simulink model "st400w_ce"  (R2016b)
settings: Solver=ode15s  StartTime=0.0  StopTime=20000  MaxStep=Ts*5  RelTol=1e-2  EnableMultiTasking=on
StopFcn:
  | %qpOASES_sequence('c');
values from neighbouring files (symbols this model uses):
  Ao = Ad    [cold_end_script.m]    (also in observateur.m = [A Bunc; zeros(size(Bunc,2),size(A,1)), eye(size(Bunc,2))])
  Aoe = Ao-L*Co    [cold_end_script.m]    (also in observateur.m)
  Boe = [Bo-L*Do Fo-L*Go L]    [cold_end_script.m]    (also in observateur.m = [Bo-L*Do L])
  Co = Cd    [cold_end_script.m]    (also in observateur.m = [C Dunc])
  Coe = eye(length(Ao))    [cold_end_script.m]    (also in observateur.m)
  Do = Dd    [cold_end_script.m]    (also in observateur.m = D)
  Doe = zeros(size(Coe*Boe))    [cold_end_script.m]    (also in observateur.m)
  Go = Gd    [cold_end_script.m]
  ini = 0    [cold_end_script.m]
  mpc = cstr_func(mpc)    [cold_end_script.m]    (also in mpc_control.m = def_pb_mpc(u_t,w_t,x_t,y_ref_t,u_ref_t,mpc))
  Tp = 5    [cold_end_script.m]
undefined symbols (not defined in the file or in its folder): mpc_control
libraries: simCryogenics_lib x36, nesl_utility x24
settings Model: Creator=FB229602  LastModifiedBy=trinhvv-admin
settings SolverCC: InitialStep=2.5
settings DataIOCC: LimitDataPoints=on  SaveFormat=Array
settings OptimizationCC: LifeSpan=inf
settings DebuggingCC: SFUnexpectedBacktrackingDiag=warning  SFNoUnconditionalDefaultTransitionDiag=warning  SFExecutionAtInitializationDiag=none
settings HardwareCC: ProdBitPerPointer=32  ProdBitPerSizeT=32  ProdBitPerPtrDiffT=32  ProdLargestAtomicFloat=None  ProdIntDivRoundTo=Undefined  ProdEndianess=Unspecified  ProdWordSize=32  ProdHWDeviceType=32-bit Generic
settings ModelReferenceCC: PropagateSignalLabelsOutOfModel=off
settings GRTTargetCC: TargetLangStandard=C89/C90 (ANSI)  GeneratePreprocessorConditionals=Disable all
settings ConfigComp: CovMetricSettings=dw  CovHtmlReporting=on  CovSaveCumulativeToWorkspaceVar=on  CovSaveSingleToWorkspaceVar=on  CovExternalEMLEnable=off
settings SimscapeCC: SimscapeLogType=all  SimscapeLogLimitData=off

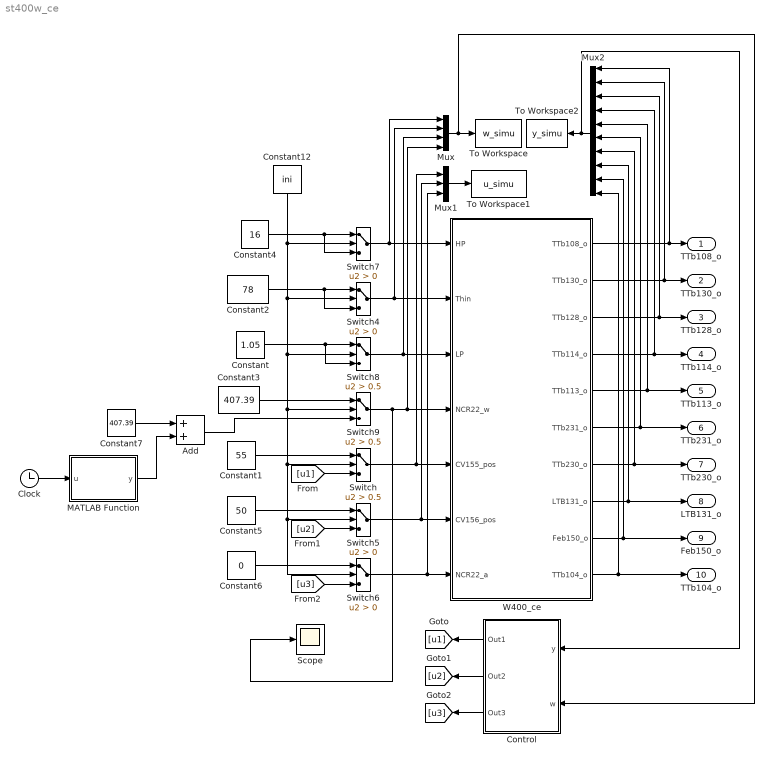
== system st400w_ce ==
  Add : Sum
  Clock : Clock
  Constant : Constant  Value=1.05
  Constant1 : Constant  Value=55
  Constant12 : Constant  Value=ini
  Constant2 : Constant  Value=78
  Constant3 : Constant  Value=407.39
  Constant4 : Constant  Value=16
  Constant5 : Constant  Value=50
  Constant6 : Constant  Value=0
  Constant7 : Constant  Value=407.39
  Control : Subsystem
  MATLAB Function : MATLAB Function  TreatAsAtomicUnit=on
  Mux : Mux
  Mux1 : Mux  Inputs=3
  Mux2 : Mux  Inputs=10
  Scope : Scope
  Switch : Switch  Criteria=u2 > Threshold  Threshold=0.5
  Switch{4..7} (4 alike) : Switch  Criteria=u2 > Threshold
  Switch8 : Switch  Criteria=u2 > Threshold  Threshold=0.5
  Switch9 : Switch  Criteria=u2 > Threshold  Threshold=0.5
  To Workspace : ToWorkspace  VariableName=w_simu  SampleTime=-1
      settings: Save2DSignal=2-D array (concatenate along first dimension)
  To Workspace1 : ToWorkspace  VariableName=u_simu  SampleTime=-1
      settings: Save2DSignal=2-D array (concatenate along first dimension)
  To Workspace2 : ToWorkspace  VariableName=y_simu  SampleTime=-1
      settings: Save2DSignal=2-D array (concatenate along first dimension)
  W400_ce : Subsystem
  TTb108_o : Outport
  TTb130_o : Outport  Port=2
  TTb128_o : Outport  Port=3
  TTb114_o : Outport  Port=4
  TTb113_o : Outport  Port=5
  TTb231_o : Outport  Port=6
  TTb230_o : Outport  Port=7
  LTB131_o : Outport  Port=8
  Feb150_o : Outport  Port=9
  TTb104_o : Outport  Port=10
  wires:
  Switch8/1 -> Mux/3, W400_ce/3(LP)
  Switch7/1 -> Mux/1, W400_ce/1(HP)
  Switch5/1 -> Mux1/2, W400_ce/6(CV156_pos)
  Switch/1 -> Mux1/1, W400_ce/5(CV155_pos)
  Switch6/1 -> Mux1/3, W400_ce/7(NCR22_a)
  W400_ce/1(TTb108_o) -> Mux2/1, TTb108_o/1
  W400_ce/2(TTb130_o) -> Mux2/2, TTb130_o/1
  W400_ce/3(TTb128_o) -> Mux2/3, TTb128_o/1
  W400_ce/4(TTb114_o) -> Mux2/4, TTb114_o/1
  W400_ce/5(TTb113_o) -> Mux2/5, TTb113_o/1
  W400_ce/6(TTb231_o) -> Mux2/6, TTb231_o/1
  W400_ce/7(TTb230_o) -> Mux2/7, TTb230_o/1
  W400_ce/8(LTB131_o) -> Mux2/8, LTB131_o/1
  W400_ce/9(Feb150_o) -> Mux2/9, Feb150_o/1
  Switch9/1 -> Scope/1, W400_ce/4(NCR22_w), Mux/4
  W400_ce/10(TTb104_o) -> TTb104_o/1, Mux2/10
  Switch4/1 -> Mux/2, W400_ce/2(Thin)
  Constant6/1 -> Switch6/1
  Constant1/1 -> Switch/1
  Constant5/1 -> Switch5/1
  Constant12/1 -> Switch6/2, Switch5/2, Switch/2, Switch9/2, Switch8/2, Switch4/2, Switch7/2
  Constant2/1 -> Switch4/3, Switch4/1
  Constant4/1 -> Switch7/3, Switch7/1
  Control/1(Out1) -> [u1]
  Control/2(Out2) -> [u2]
  Control/3(Out3) -> [u3]
  Constant/1 -> Switch8/3, Switch8/1
  Add/1 -> Switch9/3
  Mux1/1 -> To Workspace1/1
  Mux/1 -> Control/2(w), To Workspace/1
  Mux2/1 -> Control/1(y), To Workspace2/1
  [u1] -> Switch/3
  [u2] -> Switch5/3
  [u3] -> Switch6/3
  Constant3/1 -> Switch9/1
  Constant7/1 -> Add/1
  MATLAB Function/1(y) -> Add/2
  Clock/1 -> MATLAB Function/1(u)

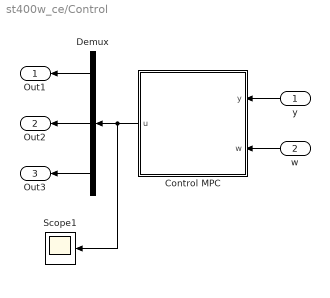
== system st400w_ce/Control ==
  y : Inport
  w : Inport  Port=2
  Control MPC : Subsystem
  Demux : Demux  Outputs=3
  Scope1 : Scope
  Out1 : Outport
  Out2 : Outport  Port=2
  Out3 : Outport  Port=3
  wires:
  Demux/1 -> Out1/1
  Demux/2 -> Out2/1
  Demux/3 -> Out3/1
  Control MPC/1(u) -> Scope1/1, Demux/1
  y/1 -> Control MPC/1(y)
  w/1 -> Control MPC/2(w)

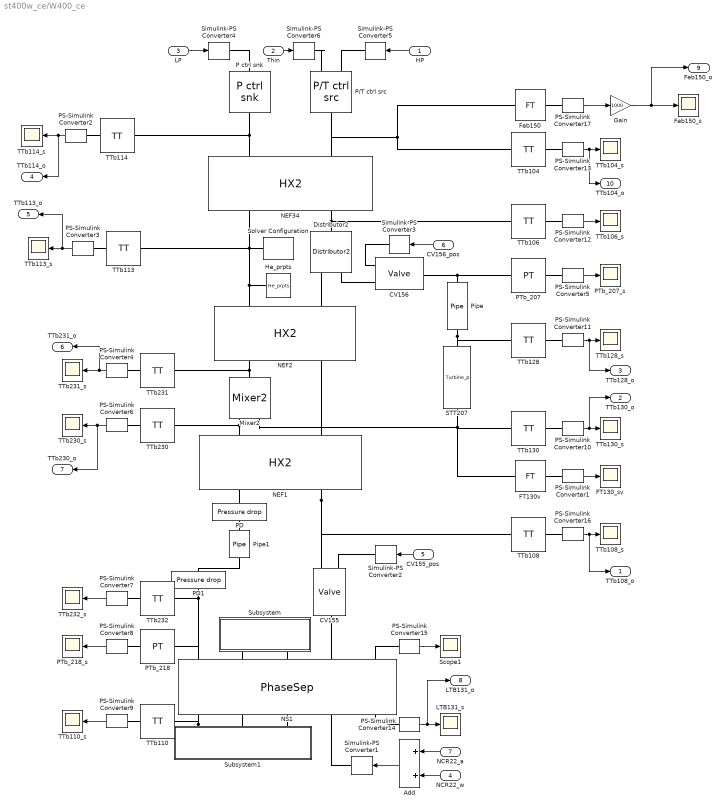
== system st400w_ce/W400_ce ==
  HP : Inport
  Thin : Inport  Port=2
  LP : Inport  Port=3
  NCR22_w : Inport  Port=4
  CV155_pos : Inport  Port=5
  CV156_pos : Inport  Port=6
  NCR22_a : Inport  Port=7
  Add : Sum
  CV155 : simCryogenics_lib/Elements/Valve  CVmax=0.55  ControlInputMin=0  ControlInputMax=100  Xt=0.86  Rv=10  lin_v=0  lim_v=0  K=2.4e-5 m^1.50000*kg^0.50000/s/bar^0.50000  Cmd_specify=off  Cmd_priority=High  Cmd=0  gamma_specify=off  gamma_priority=High  gamma=0  rho_specify=off  rho_priority=High  rho=0 kg/m^3  Xc_specify=off  Xc_priority=High  Xc=0  X_specify=off  X_priority=High  X=0  Y_specify=off  Y_priority=High  Y=0  CV_specify=off  CV_priority=High  CV=0
  CV156 : simCryogenics_lib/Elements/Valve  CVmax=Cv  ControlInputMin=0  ControlInputMax=100  Xt=0.86  Rv=Rv  lin_v=0  lim_v=0  K=2.4e-5 m^1.50000*kg^0.50000/s/bar^0.50000  Cmd_specify=off  Cmd_priority=High  Cmd=0  gamma_specify=off  gamma_priority=High  gamma=0  rho_specify=off  rho_priority=High  rho=0 kg/m^3  Xc_specify=off  Xc_priority=High  Xc=0  X_specify=off  X_priority=High  X=0  Y_specify=off  Y_priority=High  Y=0  CV_specify=off  CV_priority=High  CV=0
  Distributor2 : simCryogenics_lib/Elements/Distributor2
  FT130_sv : Scope
  FT130v : simCryogenics_lib/Sensors/FT
  Feb150 : simCryogenics_lib/Sensors/FT
  Feb150_s : Scope
  Gain : Gain  Gain=1000
  He_prpts : simCryogenics_lib/Utilities/He_prpts  P_min=0.25 bar  P_max=18 bar  T_min=2 K  T_max=80 K  N=100  Mol=4.0026 * 10 ^ (- 3) kg/mol
  LTB131_s : Scope
  Mixer2 : simCryogenics_lib/Elements/Mixer2
  NEF1 : simCryogenics_lib/Elements/HX2  N=3  Vh=2.3e-3 m^3  Vc=2.3e-3 m^3  M=13 kg  Kh=0.6 s*bar/kg  Kc=0.35 s*bar/kg  h=H1 J/s/K  Th0=10 K  Ph0=16 bar  Mh0=0.037 kg/s  Tc0=4.5 K  Pc0=1.1 bar  Mc0=0.037 kg/s
  NEF2 : simCryogenics_lib/Elements/HX2  N=3  Vh=0.02 m^3  Vc=0.03 m^3  M=100 kg  Kh=0.6 s*bar/kg  Kc=0.35 s*bar/kg  h=H2 J/s/K  Th0=20 K  Ph0=16 bar  Mh0=0.037 kg/s  Tc0=10 K  Pc0=1.1 bar  Mc0=0.037 kg/s
  NEF34 : simCryogenics_lib/Elements/HX2  N=3  Vh=0.1 m^3  Vc=0.3 m^3  M=400 kg  Kh=0.6 s*bar/kg  Kc=0.35 s*bar/kg  h=H3 J/s/K  Th0=80 K  Ph0=16 bar  Mh0=0.037 kg/s  Tc0=20 K  Pc0=1.1 bar  Mc0=0.037 kg/s
  NS1 : simCryogenics_lib/Elements/PhaseSep  Ideal1=1  DeltaT1=0.05 K  N1=10  h1=400 W/K  Ideal2=1  DeltaT2=0.05 K  N2=10  h2=400 W/K  hmax=0.8 m  S=0.1662 m^2  P0=1.2 bar  h0=62  T0=4.5 K
  P ctrl snk : simCryogenics_lib/Sources_Sinks/P ctrl snk
  P/T ctrl src : simCryogenics_lib/Sources_Sinks/P//T ctrl src
  PD : simCryogenics_lib/Utilities/Pressure drop  K=0.01/0.03 s*bar/kg
  PD1 : simCryogenics_lib/Utilities/Pressure drop  K=0.0001/0.03 s*bar/kg
  PS-Simulink Converter{1..17} (17 alike) : nesl_utility/PS-Simulink Converter  PhysicalDomain=network_engine_domain  SubClassName=ps_output  LeftPortType=input  RightPortType=output  PseudoPeriodic=off  Frequencies=[]  Unit=1  AffineConversion=off
  PTb_207 : simCryogenics_lib/Sensors/PT
  PTb_207_s : Scope
  PTb_218 : simCryogenics_lib/Sensors/PT
  PTb_218_s : Scope
  Pipe : simCryogenics_lib/Elements/Pipe  Vol=0.05 m^3  Ideal=0  P0=14 bar  T0=22 K
  Pipe1 : simCryogenics_lib/Elements/Pipe  Vol=0.162*0.3 m^3  Ideal=0  P0=1.2 bar  T0=4.5 K
  STT207 : simCryogenics_lib/Elements/Turbine_p  A=5.4278e-06 m^2  D=0.022 m  Mass=0.02 kg  cst_eff=1  eta0=0.75  Tin0=20 K  Pin0=16 bar  Pout0=1.2 bar  N0=2500 1/s  Q0=0 W  v0=0  I=0 kg*m^2  gamma_specify=off  gamma_priority=High  gamma=0  C_specify=off  C_priority=High  C=0  Z_specify=off  Z_priority=High  Z=0  Cp_specify=off  Cp_priority=High  Cp=0 kJ/kg/K  Sin_specify=off  Sin_priority=High  Sin=0 kJ/kg  T_specify=off  T_priority=High  T=0 K  HoutIs_specify=off  HoutIs_priority=High  HoutIs=0 kJ/kg  u1_specify=off  u1_priority=High  u1=0 m/s  c1_specify=off  c1_priority=High  c1=0 m/s  v_specify=off  v_priority=High  v=0  eta_specify=off  eta_priority=High  eta=0  eta_var_specify=off  eta_var_priority=High  eta_var=0  N_specify=off  N_priority=High  N=0 rad/s  Q_specify=off  Q_priority=High  Q=0 W
  Scope1 : Scope
  Simulink-PS Converter{1,3..5} (4 alike) : nesl_utility/Simulink-PS Converter  PhysicalDomain=network_engine_domain  SubClassName=ps_input  LeftPortType=input  RightPortType=output  PseudoPeriodic=off  Frequencies=[]  NoiseDistribution=none  NoiseParameters=[]  Unit=1  AffineConversion=off  InputFiltering=off  SimscapeFilterOrder=1  InputFilterTimeConstant=1  UdotUserProvided=1
  Simulink-PS Converter2 : nesl_utility/Simulink-PS Converter  PhysicalDomain=network_engine_domain  SubClassName=ps_input  LeftPortType=input  RightPortType=output  PseudoPeriodic=off  Frequencies=[]  NoiseDistribution=none  NoiseParameters=[]  Unit=1  AffineConversion=off  InputFiltering=off  SimscapeFilterOrder=1  InputFilterTimeConstant=0.001  UdotUserProvided=1
  Simulink-PS Converter6 : nesl_utility/Simulink-PS Converter  PhysicalDomain=network_engine_domain  SubClassName=ps_input  LeftPortType=input  RightPortType=output  PseudoPeriodic=off  Frequencies=[]  NoiseDistribution=none  NoiseParameters=[]  Unit=1  AffineConversion=off  InputFiltering=off  SimscapeFilterOrder=1  InputFilterTimeConstant=0.001  UdotUserProvided=1
  Solver Configuration : nesl_utility/Solver Configuration  PhysicalDomain=network_engine_domain  SubClassName=solver  LeftPortType=input  RightPortType=generic  Accelerate=off  Tones=[]  Harmonics=[]  SimulateNoise=off  Profile=off  UseLocalSampling=off  EnableSwitchedLinearOptims=on  FrequencyDomain=off  UseCCode=off  RelTol=0.001  AbsTol=1e-06  MinStep=1e-09  ToWorkspace=off  RevertToSquareIcSolve=off  NumHomotopyIterations=100  PhasorMode=off  PhasorModeNumHarmonics=1  OverrideAbsTol=off  DoDC=off  ResidualTolerance=1e-09  UseLocalSolver=off  LocalSolverChoice=NE_BACKWARD_EULER_ADVANCER  LocalSolverSampleTime=5  DoFixedCost=off  MaxNonlinIter=3  MaxModeIter=2  LinearAlgebra=Sparse  DelaysMemoryBudget=1024  AutomaticFiltering=on  FilteringTimeConstant=0.001
  Subsystem : Subsystem
  Subsystem1 : Subsystem
  TTb{104,106,108,110,113..114,128,130,230..232} (11 alike) : simCryogenics_lib/Sensors/TT
  TTb104_s : Scope
  TTb106_s : Scope
  TTb108_s : Scope
  TTb110_s : Scope
  TTb113_s : Scope
  TTb114_s : Scope
  TTb128_s : Scope
  TTb130_s : Scope
  TTb230_s : Scope
  TTb231_s : Scope
  TTb232_s : Scope
  TTb108_o : Outport
  TTb130_o : Outport  Port=2
  TTb128_o : Outport  Port=3
  TTb114_o : Outport  Port=4
  TTb113_o : Outport  Port=5
  TTb231_o : Outport  Port=6
  TTb230_o : Outport  Port=7
  LTB131_o : Outport  Port=8
  Feb150_o : Outport  Port=9
  TTb104_o : Outport  Port=10
  wires:
  Gain/1 -> Feb150_o/1, Feb150_s/1
  CV155_pos/1 -> Simulink-PS Converter2/1
  HP/1 -> Simulink-PS Converter5/1
  Thin/1 -> Simulink-PS Converter6/1
  LP/1 -> Simulink-PS Converter4/1
  NCR22_w/1 -> Add/2
  NCR22_a/1 -> Add/1
  PS-Simulink Converter17/1 -> Gain/1
  PS-Simulink Converter16/1 -> TTb108_o/1, TTb108_s/1
  PS-Simulink Converter1/1 -> FT130_sv/1
  CV156_pos/1 -> Simulink-PS Converter3/1
  PS-Simulink Converter5/1 -> PTb_207_s/1
  PS-Simulink Converter12/1 -> TTb106_s/1
  PS-Simulink Converter11/1 -> TTb128_o/1, TTb128_s/1
  PS-Simulink Converter10/1 -> TTb130_o/1, TTb130_s/1
  PS-Simulink Converter9/1 -> TTb110_s/1
  PS-Simulink Converter8/1 -> PTb_218_s/1
  PS-Simulink Converter7/1 -> TTb232_s/1
  PS-Simulink Converter6/1 -> TTb230_o/1, TTb230_s/1
  PS-Simulink Converter4/1 -> TTb231_o/1, TTb231_s/1
  PS-Simulink Converter3/1 -> TTb113_o/1, TTb113_s/1
  PS-Simulink Converter2/1 -> TTb114_s/1, TTb114_o/1
  PS-Simulink Converter15/1 -> Scope1/1
  PS-Simulink Converter14/1 -> LTB131_o/1, LTB131_s/1
  Add/1 -> Simulink-PS Converter1/1
  PS-Simulink Converter13/1 -> TTb104_o/1, TTb104_s/1
  connections:
  Simulink-PS Converter6/RConn1 -- P/T ctrl src/LConn2
  Simulink-PS Converter5/RConn1 -- P/T ctrl src/LConn1
  He_prpts/RConn1 -- Solver Configuration/RConn1 -- TTb113/LConn1 -- NEF34/RConn1 -- NEF2/LConn1
  Simulink-PS Converter4/RConn1 -- P ctrl snk/LConn1
  Pipe1/LConn1 -- PD1/RConn1
  Pipe1/RConn1 -- PD/LConn1
  Feb150/RConn1 -- PS-Simulink Converter17/LConn1
  PS-Simulink Converter4/LConn1 -- TTb231/RConn1
  Subsystem1/RConn2 -- NS1/RConn2
  PS-Simulink Converter7/LConn1 -- TTb232/RConn1
  TTb104/RConn1 -- PS-Simulink Converter13/LConn1
  TTb106/RConn1 -- PS-Simulink Converter12/LConn1
  Simulink-PS Converter3/RConn1 -- CV156/LConn1
  PS-Simulink Converter6/LConn1 -- TTb230/RConn1
  TTb128/RConn1 -- PS-Simulink Converter11/LConn1
  PS-Simulink Converter10/LConn1 -- TTb130/RConn1
  PS-Simulink Converter2/LConn1 -- TTb114/RConn1
  PS-Simulink Converter8/LConn1 -- PTb_218/RConn1
  PS-Simulink Converter5/LConn1 -- PTb_207/RConn1
  Subsystem1/RConn3 -- NS1/RConn3
  PS-Simulink Converter15/LConn1 -- NS1/LConn5
  PD/RConn1 -- NEF1/RConn1
  PS-Simulink Converter16/LConn1 -- TTb108/RConn1
  PS-Simulink Converter14/LConn1 -- NS1/RConn5
  Simulink-PS Converter1/RConn1 -- NS1/RConn4
  Distributor2/RConn2 -- NEF2/LConn2
  Simulink-PS Converter2/RConn1 -- CV155/LConn1
  NS1/LConn4 -- CV155/RConn1
  PS-Simulink Converter9/LConn1 -- TTb110/RConn1
  FT130v/RConn1 -- PS-Simulink Converter1/LConn1
  NEF2/RConn2 -- NEF1/LConn2
  Distributor2/RConn1 -- CV156/LConn2
  Subsystem/RConn2 -- NS1/LConn3
  Subsystem/RConn1 -- NS1/LConn2
  PS-Simulink Converter3/LConn1 -- TTb113/RConn1
  NS1/RConn1 -- Subsystem1/RConn1 -- TTb110/LConn1
  TTb104/LConn1 -- P/T ctrl src/RConn1 -- NEF34/LConn2 -- Feb150/LConn1
  TTb114/LConn1 -- P ctrl snk/RConn1 -- NEF34/LConn1
  NEF1/LConn1 -- TTb230/LConn1 -- Mixer2/LConn1
  Mixer2/LConn2 -- TTb130/LConn1 -- FT130v/LConn1 -- STT207/RConn1
  NEF2/RConn1 -- TTb231/LConn1 -- Mixer2/RConn1
  Distributor2/LConn1 -- TTb106/LConn1 -- NEF34/RConn2
  CV156/RConn1 -- PTb_207/LConn1 -- Pipe/LConn1
  STT207/LConn1 -- TTb128/LConn1 -- Pipe/RConn1
  NEF1/RConn2 -- CV155/LConn2 -- TTb108/LConn1
  TTb232/LConn1 -- PD1/LConn1 -- NS1/LConn1 -- PTb_218/LConn1

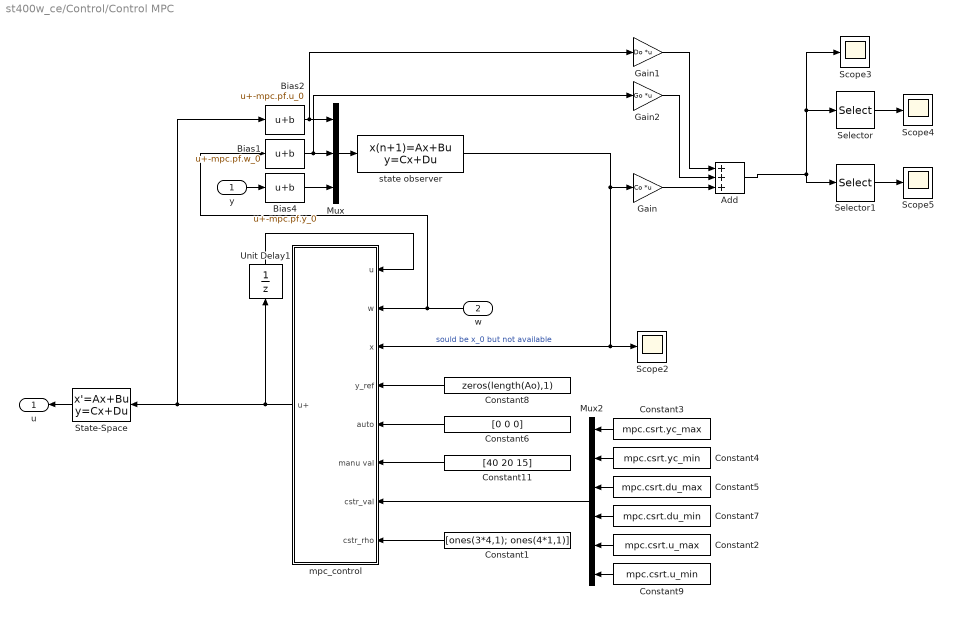
== system st400w_ce/Control/Control MPC ==
  y : Inport
  w : Inport  Port=2
  Add : Sum  Inputs=3
  Bias1 : Bias  Bias=-mpc.pf.w_0
  Bias2 : Bias  Bias=-mpc.pf.u_0
  Bias4 : Bias  Bias=-mpc.pf.y_0
  Constant1 : Constant  Value=[ones(3*4,1); ones(4*1,1)]
  Constant11 : Constant  Value=[40 20 15]
  Constant2 : Constant  Value=mpc.csrt.u_max
  Constant3 : Constant  Value=mpc.csrt.yc_max
  Constant4 : Constant  Value=mpc.csrt.yc_min
  Constant5 : Constant  Value=mpc.csrt.du_max
  Constant6 : Constant  Value=[0 0 0]
  Constant7 : Constant  Value=mpc.csrt.du_min
  Constant8 : Constant  Value=zeros(length(Ao),1)
  Constant9 : Constant  Value=mpc.csrt.u_min
  Gain : Gain  Gain=Co  Multiplication=Matrix(K*u)
  Gain1 : Gain  Gain=Do  Multiplication=Matrix(K*u)
  Gain2 : Gain  Gain=Go  Multiplication=Matrix(K*u)
  Mux : Mux  Inputs=3
  Mux2 : Mux  Inputs=6
  Scope{2..5} (4 alike) : Scope
  Selector : Selector  IndexOptions=Index vector (dialog)  Indices=8  OutputSizes=1
  Selector1 : Selector  IndexOptions=Index vector (dialog)  Indices=2  OutputSizes=1
  State-Space : StateSpace  A=-diag([100 100 100])  B=diag([100 100 100])  C=eye(3)  D=zeros(3)  X0=mpc.pf.u_0
  Unit Delay1 : UnitDelay  InitialCondition=mpc.pf.u_0  SampleTime=Tp
  mpc_control : Subsystem
  state observer : DiscreteStateSpace  A=Aoe  B=Boe  C=Coe  D=Doe  SampleTime=Tp
  u : Outport  PortDimensions=3
  wires:
  Unit Delay1/1 -> mpc_control/1(u)
  Constant8/1 -> mpc_control/4(y_ref)
  Constant6/1 -> mpc_control/5(auto)
  Constant1/1 -> mpc_control/8(cstr_rho)
  Constant11/1 -> mpc_control/6(manu val)
  State-Space/1 -> u/1
  Mux/1 -> state observer/1
  Bias1/1 -> Gain2/1, Mux/2
  Bias2/1 -> Gain1/1, Mux/1
  state observer/1 -> mpc_control/3(x), Scope2/1, Gain/1  "sould be x_0 but not available"
  Constant3/1 -> Mux2/1
  Constant4/1 -> Mux2/2
  Constant2/1 -> Mux2/5
  Constant9/1 -> Mux2/6
  Constant5/1 -> Mux2/3
  Constant7/1 -> Mux2/4
  mpc_control/1(u+) -> Unit Delay1/1, Bias2/1, State-Space/1
  Mux2/1 -> mpc_control/7(cstr_val)
  w/1 -> mpc_control/2(w), Bias1/1
  y/1 -> Bias4/1
  Bias4/1 -> Mux/3
  Gain/1 -> Add/3
  Gain2/1 -> Add/2
  Gain1/1 -> Add/1
  Selector/1 -> Scope4/1
  Add/1 -> Scope3/1, Selector/1, Selector1/1
  Selector1/1 -> Scope5/1

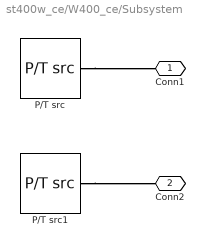
== system st400w_ce/W400_ce/Subsystem ==
  P/T src : simCryogenics_lib/Sources_Sinks/P//T src  P=1 bar  T=300 K
  P/T src1 : simCryogenics_lib/Sources_Sinks/P//T src  P=1 bar  T=300 K
  Conn1 : PMIOPort  Port=1  Side=Right
  Conn2 : PMIOPort  Port=2  Side=Right
  connections:
  P/T src/RConn1 -- Conn1/RConn1
  P/T src1/RConn1 -- Conn2/RConn1

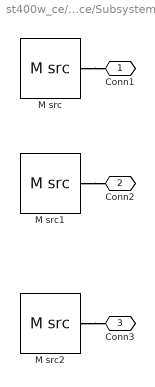
== system st400w_ce/W400_ce/Subsystem1 ==
  M src : simCryogenics_lib/Sources_Sinks/M src  M=0 kg/s
  M src1 : simCryogenics_lib/Sources_Sinks/M src  M=0 kg/s
  M src2 : simCryogenics_lib/Sources_Sinks/M src  M=0 kg/s
  Conn1 : PMIOPort  Port=1  Side=Right
  Conn2 : PMIOPort  Port=2  Side=Right
  Conn3 : PMIOPort  Port=3  Side=Right
  connections:
  M src/RConn1 -- Conn1/RConn1
  M src1/RConn1 -- Conn2/RConn1
  M src2/RConn1 -- Conn3/RConn1

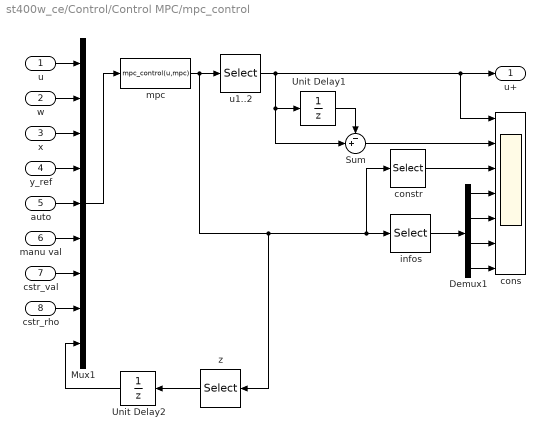
== system st400w_ce/Control/Control MPC/mpc_control ==
  u : Inport
  w : Inport  Port=2
  x : Inport  Port=3
  y_ref : Inport  Port=4
  auto : Inport  Port=5
  manu val : Inport  Port=6
  cstr_val : Inport  Port=7
  cstr_rho : Inport  Port=8
  Demux1 : Demux
  Mux1 : Mux  Inputs=9
  Sum : Sum  Inputs=-+|
  Unit Delay1 : UnitDelay  InitialCondition=zeros(3,1)  SampleTime=Tp
  Unit Delay2 : UnitDelay  InitialCondition=zeros(length(mpc.pb.H),1)  SampleTime=Tp
  cons : Scope  NumInputPorts=7
  constr : Selector  IndexOptions=Index vector (dialog)  Indices=4:6  OutputSizes=1
  infos : Selector  IndexOptions=Index vector (dialog)  Indices=7:10  OutputSizes=1
  mpc : MATLABFcn  MATLABFcn=mpc_control(u,mpc)  OutputDimensions=length(mpc.pb.H)+10+3  OutputSignalType=real  Output1D=off  SampleTime=Tp
  u1..2 : Selector  IndexOptions=Index vector (dialog)  Indices=1:3  OutputSizes=1
  z : Selector  IndexOptions=Index vector (dialog)  Indices=11:11+size(mpc.pb.H)-1  OutputSizes=1
  u+ : Outport  PortDimensions=3
  wires:
  u1..2/1 -> cons/1, u+/1, Sum/2, Unit Delay1/1
  infos/1 -> Demux1/1
  u/1 -> Mux1/1
  auto/1 -> Mux1/5
  y_ref/1 -> Mux1/4
  x/1 -> Mux1/3
  w/1 -> Mux1/2
  Mux1/1 -> mpc/1
  Unit Delay1/1 -> Sum/1
  Demux1/4 -> cons/7
  Demux1/3 -> cons/6
  Demux1/2 -> cons/5
  Demux1/1 -> cons/4
  constr/1 -> cons/3
  Sum/1 -> cons/2
  manu val/1 -> Mux1/6
  cstr_rho/1 -> Mux1/8
  cstr_val/1 -> Mux1/7
  mpc/1 -> u1..2/1, infos/1, constr/1, z/1
  Unit Delay2/1 -> Mux1/9
  z/1 -> Unit Delay2/1

== matlab function st400w_ce/MATLAB Function ==
  data: u input; y output
function y=fcn(u)

u=u-1e4;         
    
y=0;
if (180<=u)&&(u<540),      y=-225;    end     
if (540<=u)&&(u<840),      y=0;     end
if (840<=u)&&(u<1020),      y=-225;        end
if (1020<=u)&&(u<1200),      y=0;    end     
if (1200<=u)&&(u<1380),      y=-50;     end
if (1380<=u),      y=0;        end
